simulink model "Four_compartment_TOP"  (R2019b)
settings: Solver=VariableStepAuto  StartTime=0.0  StopTime=time  RelTol=1e-3
values from neighbouring files (symbols this model uses):
  breath = 60/f    (= 4)    [Model_simulation.m]
  E1 = 10    [Model_simulation.m]
  E2 = 10    [Model_simulation.m]
  E3 = 10    [Model_simulation.m]
  E4 = 10    [Model_simulation.m]
  E_high = 100    [Model_simulation.m]
  E_th = 15    [Model_simulation.m]
  insptime = (ieratio(1)/(ieratio(1)+ieratio(2)))*100    [Model_simulation.m]
  Pcontrol = 5    [Model_simulation.m]
  PEEP = 5    [Model_simulation.m]
  R = 30    [Model_simulation.m]
  R1 = 5    [Model_simulation.m]
  R2 = 5    [Model_simulation.m]
  R3 = 5    [Model_simulation.m]
  R4 = 5    [Model_simulation.m]
  TOP1 = 0    [Model_simulation.m]
  TOP2 = 20    [Model_simulation.m]
  TOP3 = 10    [Model_simulation.m]
  TOP4 = 15    [Model_simulation.m]
  V0 = 2    [Model_simulation.m]
  V0_th = 4.6    [Model_simulation.m]
settings Model: Creator=Amne  LastModifiedBy=Amne
settings DataIOCC: ReturnWorkspaceOutputs=off
settings DebuggingCC: ArithmeticOperatorsInVariantConditions=warning
settings SFSimCC: SimUseLocalCustomCode=off  CustomCodeUndefinedFunction=UseInterfaceOnly
settings RTWCC: RTWUseLocalCustomCode=off

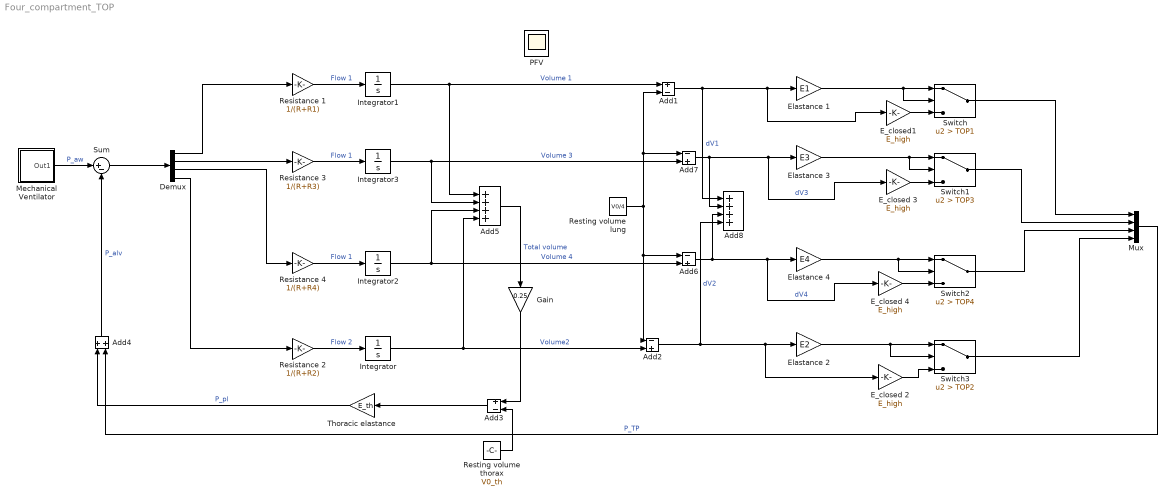
== system Four_compartment_TOP ==
  Add1 : Sum  Inputs=+-
  Add2 : Sum  Inputs=-+
  Add3 : Sum  Inputs=+-
  Add4 : Sum
  Add5 : Sum  Inputs=++++
  Add6 : Sum  Inputs=-+
  Add7 : Sum  Inputs=-+
  Add8 : Sum  Inputs=++++
  Demux : Demux
  E_closed 2 : Gain  Gain=E_high
  "E_closed 3 " : Gain  Gain=E_high
  E_closed 4 : Gain  Gain=E_high
  "E_closed1 " : Gain  Gain=E_high
  Elastance 1 : Gain  Gain=E1
  "Elastance 2 " : Gain  Gain=E2
  Elastance 3 : Gain  Gain=E3
  Elastance 4 : Gain  Gain=E4
  Gain : Gain  Gain=0.25
  Integrator{,1..3} (4 alike) : Integrator
  "Mechanical Ventilator " : Subsystem
  Mux : Mux
  Resistance 1 : Gain  Gain=1/(R+R1)
  Resistance 2 : Gain  Gain=1/(R+R2)
  Resistance 3 : Gain  Gain=1/(R+R3)
  Resistance 4 : Gain  Gain=1/(R+R4)
  "Resting volume lung " : Constant  Value=V0/4
  Resting volume thorax : Constant  Value=V0_th
  Sum : Sum  Inputs=|+-
  Switch : Switch  Criteria=u2 > Threshold  Threshold=TOP1
  Switch1 : Switch  Criteria=u2 > Threshold  Threshold=TOP3
  Switch2 : Switch  Criteria=u2 > Threshold  Threshold=TOP4
  Switch3 : Switch  Criteria=u2 > Threshold  Threshold=TOP2
  Thoracic elastance : Gain  Gain=E_th
  PFV : Scope
  wires:
  "Mechanical Ventilator "/1(Out1) -> Sum/1  "P_aw"
  Resistance 1/1 -> Integrator1/1  "Flow 1"
  Mux/1 -> Add4/2  "P_TP"
  Resting volume thorax/1 -> Add3/2
  Add3/1 -> Thoracic elastance/1
  Thoracic elastance/1 -> Add4/1  "P_pl"
  Add4/1 -> Sum/2  "P_alv"
  "Resting volume lung "/1 -> Add2/1, Add6/1, Add7/1, Add1/2
  Integrator/1 -> Add5/4, Add2/2  "Volume2"
  Sum/1 -> Demux/1
  Demux/1 -> Resistance 1/1
  Resistance 2/1 -> Integrator/1  "Flow 2"
  Integrator1/1 -> Add5/1, Add1/1  "Volume 1"
  Add5/1 -> Gain/1  "Total volume"
  Add2/1 -> Add8/4, E_closed 2/1, "Elastance 2 "/1  "dV2"
  Add1/1 -> Add8/1, "E_closed1 "/1, Elastance 1/1  "dV1"
  Demux/4 -> Resistance 2/1
  Demux/3 -> Resistance 4/1
  Resistance 4/1 -> Integrator2/1  "Flow 1"
  Integrator2/1 -> Add6/2, Add5/3  "Volume 4"
  Integrator3/1 -> Add5/2, Add7/2  "Volume 3"
  Demux/2 -> Resistance 3/1
  Resistance 3/1 -> Integrator3/1  "Flow 1"
  Add7/1 -> Add8/2, "E_closed 3 "/1, Elastance 3/1  "dV3"
  Add6/1 -> Add8/3, E_closed 4/1, Elastance 4/1  "dV4"
  Gain/1 -> Add3/1
  Elastance 1/1 -> Switch/2, Switch/1
  "E_closed1 "/1 -> Switch/3
  Switch/1 -> Mux/1
  Elastance 3/1 -> Switch1/2, Switch1/1
  Switch1/1 -> Mux/2
  "E_closed 3 "/1 -> Switch1/3
  Elastance 4/1 -> Switch2/2, Switch2/1
  Switch2/1 -> Mux/3
  E_closed 4/1 -> Switch2/3
  Switch3/1 -> Mux/4
  "Elastance 2 "/1 -> Switch3/2, Switch3/1
  E_closed 2/1 -> Switch3/3

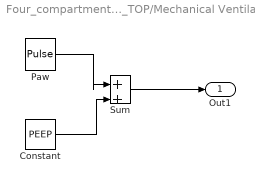
== system Four_compartment_TOP/Mechanical Ventilator  ==
  Constant : Constant  Value=PEEP  SampleTime=0.1
  Paw : DiscretePulseGenerator  PulseType=Time based  Amplitude=Pcontrol  Period=breath  PulseWidth=insptime  PhaseDelay=5  SampleTime=0.1
  Sum : Sum  Inputs=|++
  Out1 : Outport  VectorParamsAs1DForOutWhenUnconnected=off
  wires:
  Paw/1 -> Sum/1
  Constant/1 -> Sum/2
  Sum/1 -> Out1/1
